simulink model "S1_Analoger_Multiplizierer"  (Simulink 8.1)
settings: Solver=ode3  StartTime=0.0  StopTime=0.5  FixedStep=1/fs  RelTol=1e-3
values from neighbouring files (symbols this model uses):
  f1 = 400    [PLL_Parameter.m]
  f2 = 20    [PLL_Parameter.m]
  fs = fs/10    (= 100000)    [PLL_Parameter.m]
undefined symbols (not defined in the file or in its folder): get
libraries: dspspect3 x1, dspsigops x1, dspsnks4 x1
settings Model: Creator=Administrator  LastModifiedBy=felix

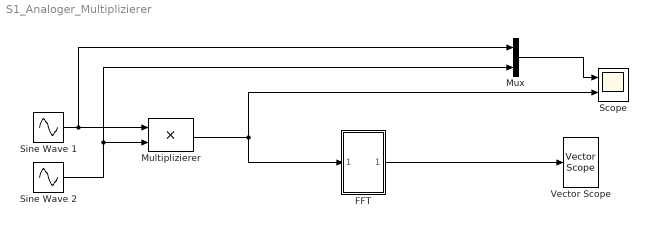
== system S1_Analoger_Multiplizierer ==
  FFT : Subsystem  mask{Buffer_Length=2^14, nfft=2^14}
      mask prompts: Buffer_Length "Buffer length?"; nfft "FFt length?"
  Multiplizierer : Product  SaturateOnIntegerOverflow=on  RndMeth=Zero  InputSameDT=on  OutDataTypeStr=Inherit: Same as first input
  Mux : Mux  Inputs=2
  Scope : Scope  NumInputPorts=2
      settings: TimeRange=0.5  YMin=-1.5~-3  YMax=1.5~3
  Sine Wave 1 : Sin  Frequency=2 * pi * f1  SampleTime=1/fs
  Sine Wave 2 : Sin  Frequency=2 * pi * f2  SampleTime=1/fs
  Vector Scope : dspsnks4/Vector Scope  ScopeProperties=on  Domain=Frequency  HorizSpan=1  DisplayProperties=off  AxisGrid=on  Memory=off  FrameNumber=on  AxisLegend=off  AxisZoom=off  OpenScopeAtSimStart=on  OpenScopeImmediately=off  FigPos=get(0,'defaultfigureposition')  AxisProperties=off  XUnits=Hertz  XRange=[0...Fs/2]  InheritXIncr=on  XIncr=1  XLabel=Time  XLimit=User-defined  XMin=0  XMax=500  XStart=0  YUnits=dB  YLabel=Amplitude  LineProperties=off  XAxisParamsVer=6.9
      settings: YMin=-100  YMax=100
  wires:
  Mux/1 -> Scope/1
  Sine Wave 2/1 -> Multiplizierer/2, Mux/2
  Sine Wave 1/1 -> Multiplizierer/1, Mux/1
  Multiplizierer/1 -> Scope/2, FFT/1(In1)
  FFT/1(Out1) -> Vector Scope/1

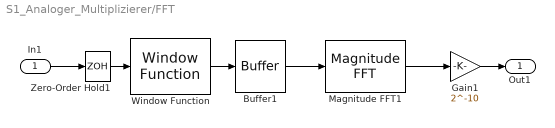
== system S1_Analoger_Multiplizierer/FFT ==
  In1 : Inport
  Buffer1 : Buffer  N=Buffer_Length  TreatMby1Signals=One channel
  Gain1 : Gain  Gain=2^-10
  Magnitude FFT1 : dspspect3/Magnitude FFT  mag_or_magsq=Magnitude squared  FFTImplementation=Auto  fftLenInherit=off  fftsize=nfft
  Window Function : dspsigops/Window Function  winmode=Apply window to input  wintype=Blackman  sampmode=Continuous  samptime=1  N=64  Rs=50  beta=10  winsamp=Symmetric  UserWindow=hamming  OptParams=off  UserParams={'symmetric'}  RowConvenienceOn=on  dataType=double  isSigned=on  wordLen=16  udDataType=sfix(16)  fracBitsMode=Best precision  numFracBits=15  roundingMode=Floor  overflowMode=off  numSidelobes=4  sidelobeLevel=-30
  Zero-Order Hold1 : ZeroOrderHold  SampleTime=1/fs
  Out1 : Outport
  wires:
  Zero-Order Hold1/1 -> Window Function/1
  Buffer1/1 -> Magnitude FFT1/1
  Magnitude FFT1/1 -> Gain1/1
  Window Function/1 -> Buffer1/1
  In1/1 -> Zero-Order Hold1/1
  Gain1/1 -> Out1/1
